simulink model "PID"  (R2020b)
settings: Solver=VariableStepAuto  StartTime=0.0  StopTime=10000  RelTol=1e-3
values from neighbouring files (symbols this model uses):
  A = [0 -theta2 0; 0 -1/theta3 1/theta3; 0 0 -1/theta3]    [script1.m]
  B = [0; 0; 1/theta3]    [script1.m]
  C = [1 0 0]    [script1.m]
  F_k = k*[1/theta2 -theta3 -theta3]    [script1.m]
undefined symbols (not defined in the file or in its folder): A_zoh, B_zoh, C_zoh, Gr, L_zoh, Ts
libraries: pid_lib x1
settings Model: Creator=Francesco  LastModifiedBy=Francesco
settings SolverCC: AlgebraicLoopSolver=LineSearch

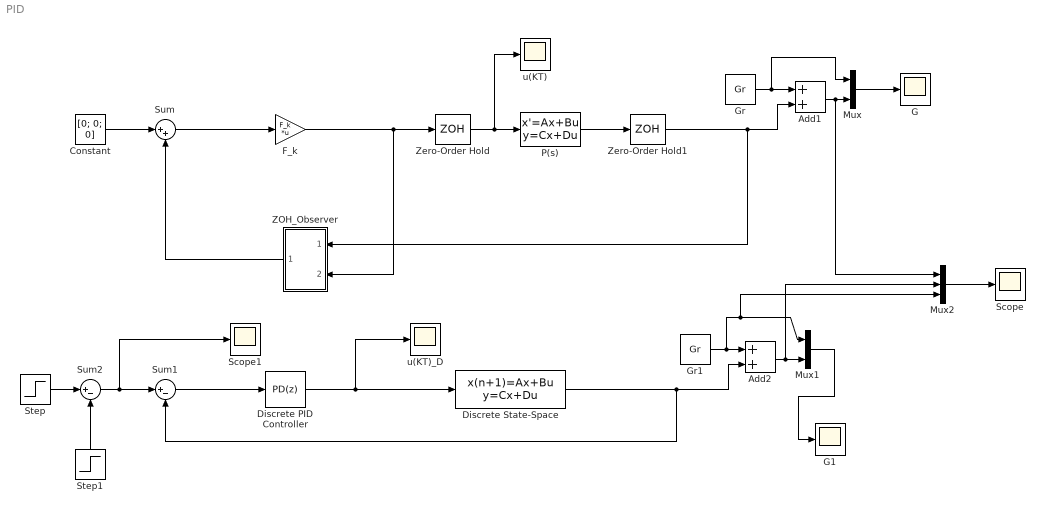
== system PID ==
  Add1 : Sum
  Add2 : Sum
  Constant : Constant  Value=[0; 0; 0]
  Discrete PID Controller : pid_lib/PID Controller  Controller=PD  Form=Parallel  TimeDomain=Discrete-time  UseExternalTs=off  SampleTime=-1  IntegratorMethod=Forward Euler  FilterMethod=Forward Euler  ControllerParametersSource=internal  P=-5.2278843413754e-05  I=-1.5815e-5  D=0  UseFilter=on  N=100  TunerSelectOption=Transfer Function Based (PID Tuner App)  InitialConditionSource=internal  InitialConditionForIntegrator=0  InitialConditionForFilter=0  DifferentiatorICPrevScaledInput=0  ExternalReset=none  TrackingMode=off  Kt=1  LimitOutput=off  SatLimitsSource=internal  UpperSaturationLimit=inf  LowerSaturationLimit=-inf  LinearizeAsGain=off  AntiWindupMode=none  Kb=1  POutMin=[]  POutMax=[]  IOutMin=[]  IOutMax=[]  DOutMin=[]  DOutMax=[]  NOutMin=[]  NOutMax=[]  SumOutMin=[]  SumOutMax=[]  SaturationOutMin=[]  SaturationOutMax=[]  PParamMin=[]  PParamMax=[]  IParamMin=[]  IParamMax=[]  DParamMin=[]  DParamMax=[]  NParamMin=[]  NParamMax=[]  KbParamMin=[]  KbParamMax=[]  KtParamMin=[]  KtParamMax=[]  KbOutMin=[]  KbOutMax=[]  KtOutMin=[]  KtOutMax=[]  IntegratorOutMin=[]  IntegratorOutMax=[]  FilterOutMin=[]  FilterOutMax=[]  SumI1OutMin=[]  SumI1OutMax=[]  SumI2OutMin=[]  SumI2OutMax=[]  SumI3OutMin=[]  SumI3OutMax=[]  SumI4OutMin=[]  SumI4OutMax=[]  SumDOutMin=[]  SumDOutMax=[]  DifferentiatorOutMin=[]  DifferentiatorOutMax=[]  FilterDiffOutCoefMin=[]  FilterDiffOutCoefMax=[]  ReciprocalOutMin=[]  ReciprocalOutMax=[]  SumDenOutMin=[]  SumDenOutMax=[]  SumNumOutMin=[]  SumNumOutMax=[]  DivideOutMin=[]  DivideOutMax=[]  UdiffTsProdOutMin=[]  UdiffTsProdOutMax=[]  NTsProdOutMin=[]  NTsProdOutMax=[]  UintegralTsProdOutMin=[]  UintegralTsProdOutMax=[]  UngainTsProdOutMin=[]  UngainTsProdOutMax=[]  IntegratorContinuousStateAttributes=''  IntegratorStateMustResolveToSignalObject=off  IntegratorRTWStateStorageClass=Auto  FilterContinuousStateAttributes=''  FilterStateMustResolveToSignalObject=off  FilterRTWStateStorageClass=Auto  ParallelPVariant=InternalParameters  IdealPVariant=Disabled  IVariant=Disabled  DVariant=InternalParameters  IntegratorVariant=Disabled  SatVariant=Disabled  AWVariant=Disabled  PCopyVariant=Disabled  TRVariant=Disabled  FdbkBlocksVariant=Forward  IdealPFdbkVariant=Disabled  SatFdbkVariant=Disabled  DerivativeFilterVariant=ForwardEulerFilter  NVariant=InternalParameters  NCopyVariant=Disabled  FilterICVariant=InternalICsFilter  IntegratorICVariant=Disabled  ExternalResetVariant=Disabled  TRSumVariant=Passthrough  SumFdbkVariant=Disabled  SumVariant=Sum_PD  TsampFilterVariant=InternalTs  TsampNgainVariant=Passthrough  TsampIntegralVariant=Disabled_SignalSpec  ExternalSaturationOutDataTypeStr=Inherit: Same as second input
  Discrete State-Space : DiscreteStateSpace  A=A_zoh  B=B_zoh  C=C_zoh  D=0  InitialCondition=[130; 0; 0]  SampleTime=-1
  F_k : Gain  Gain=F_k  Multiplication=Matrix(K*u)
  G : Scope
  G1 : Scope
  Gr : Constant  Value=Gr
  Gr1 : Constant  Value=Gr
  Mux : Mux  Inputs=2
  Mux1 : Mux  Inputs=2
  Mux2 : Mux  Inputs=3
  P(s) : StateSpace  A=A  B=B  C=C  D=0  InitialCondition=[130; 0; 0]
  Scope : Scope
  Scope1 : Scope
  Step : Step  SampleTime=0
  Step1 : Step  Time=300  SampleTime=0
  Sum : Sum  Inputs=|++
  Sum1 : Sum  Inputs=|+-
  Sum2 : Sum  Inputs=|+-
  ZOH_Observer : Subsystem
  Zero-Order Hold : ZeroOrderHold  SampleTime=Ts
  Zero-Order Hold1 : ZeroOrderHold  SampleTime=Ts
  u(KT) : Scope
  u(KT)_D : Scope
  wires:
  Constant/1 -> Sum/1
  Gr/1 -> Add1/1, Mux/1
  Zero-Order Hold/1 -> u(KT)/1, P(s)/1
  Sum/1 -> F_k/1
  ZOH_Observer/1(Out1) -> Sum/2
  Mux/1 -> G/1
  Zero-Order Hold1/1 -> ZOH_Observer/1(In1), Add1/2
  Add1/1 -> Mux2/1, Mux/2
  Sum1/1 -> Discrete PID Controller/1
  P(s)/1 -> Zero-Order Hold1/1
  F_k/1 -> ZOH_Observer/2(In2), Zero-Order Hold/1
  Discrete PID Controller/1 -> Discrete State-Space/1, u(KT)_D/1
  Mux1/1 -> G1/1
  Gr1/1 -> Add2/1, Mux2/3, Mux1/1
  Discrete State-Space/1 -> Add2/2, Sum1/2
  Add2/1 -> Mux2/2, Mux1/2
  Sum2/1 -> Scope1/1, Sum1/1
  Mux2/1 -> Scope/1
  Step/1 -> Sum2/1
  Step1/1 -> Sum2/2

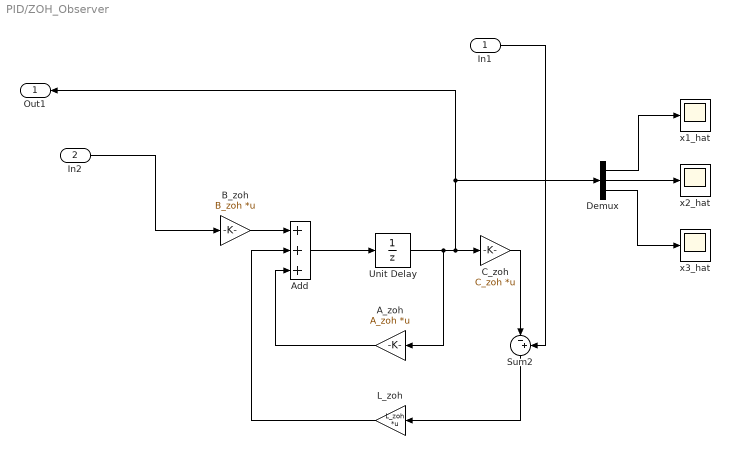
== system PID/ZOH_Observer ==
  In1 : Inport
  In2 : Inport  Port=2
  A_zoh : Gain  Gain=A_zoh  Multiplication=Matrix(K*u)
  Add : Sum  Inputs=+++
  B_zoh : Gain  Gain=B_zoh  Multiplication=Matrix(K*u)
  C_zoh : Gain  Gain=C_zoh  Multiplication=Matrix(K*u)
  Demux : Demux  Outputs=3
  L_zoh : Gain  Gain=L_zoh  Multiplication=Matrix(K*u)
  Sum2 : Sum  Inputs=|-+
  Unit Delay : UnitDelay  SampleTime=-1  HasFrameUpgradeWarning=on
  x1_hat : Scope
  x2_hat : Scope
  x3_hat : Scope
  Out1 : Outport
  wires:
  In1/1 -> Sum2/2
  B_zoh/1 -> Add/1
  Sum2/1 -> L_zoh/1
  L_zoh/1 -> Add/2
  C_zoh/1 -> Sum2/1
  A_zoh/1 -> Add/3
  Add/1 -> Unit Delay/1
  In2/1 -> B_zoh/1
  Demux/1 -> x1_hat/1
  Unit Delay/1 -> A_zoh/1, Demux/1, Out1/1, C_zoh/1
  Demux/2 -> x2_hat/1
  Demux/3 -> x3_hat/1
